simulink model "uas_main_latest"  (R2025a)
settings: Solver=FixedStepAuto  StartTime=0.0  StopTime=Inf  FixedStep=sample_time  RelTol=1e-3
model workspace: external: MAT-File (data not in the file)
values from neighbouring files (symbols this model uses):
  arm_length = 0.17    [test_uas_parameters.m]    (also in uas_parameters.m; uas_parameters_akin.m; uas_parameters_brushless.m = 0.046)
  drag_coefficient = 0.47    [uas_parameters.m]    (also in uas_parameters_akin.m; uas_parameters_brushless.m)
  g = 9.80665    [test_uas_parameters.m]    (also in uas_parameters.m; uas_parameters_akin.m; uas_parameters_brushless.m)
  inertia_xx = 0.007    [test_uas_parameters.m]    (also in uas_parameters.m; uas_parameters_akin.m; uas_parameters_brushless.m = 1.657171e-05)
  inertia_yy = 0.007    [test_uas_parameters.m]    (also in uas_parameters.m; uas_parameters_akin.m; uas_parameters_brushless.m = 1.6655602e-05)
  inertia_zz = 0.012    [test_uas_parameters.m]    (also in uas_parameters.m; uas_parameters_akin.m; uas_parameters_brushless.m = 2.9261652e-05)
  mass_drone = 0.68    [test_uas_parameters.m]    (also in uas_parameters.m; uas_parameters_akin.m; uas_parameters_brushless.m = 0.037)
  mass_total = mass_drone    (= 0.68)    [test_uas_parameters.m]    (also in uas_parameters.m; uas_parameters_akin.m; uas_parameters_brushless.m = 0.037)
  max_rot_velocity = 838    [uas_parameters.m]    (also in uas_parameters_akin.m; uas_parameters_brushless.m)
  mix_matrix = inv(motor_constant * allocation_matrix)    [test_uas_parameters.m]    (also in uas_parameters.m; uas_parameters_akin.m; uas_parameters_brushless.m)
  moment_constant = 0.016    [test_uas_parameters.m]    (also in uas_parameters.m; uas_parameters_akin.m; uas_parameters_brushless.m = 0.006)
  motor_constant = 8.54858e-06    [test_uas_parameters.m]    (also in uas_parameters.m; uas_parameters_akin.m; uas_parameters_brushless.m = 1.45e-08)
  publish_rate = sample_time    (= 0.04)    [test_uas_parameters.m]    (also in uas_parameters.m; uas_parameters_akin.m; uas_parameters_brushless.m)
  reference_area = pi * (75e-3)^2    (= 0.0176714586764)    [uas_parameters.m]    (also in uas_parameters_akin.m; uas_parameters_brushless.m)
  rotor_offset_top = 0.01    [uas_parameters.m]    (also in uas_parameters_akin.m; uas_parameters_brushless.m)
  route = route_scaled    [generate_route_for_simulink.m]    (also in uas_parameters.m = route_smooth; uas_parameters_akin.m = route_dense; uas_parameters_brushless.m = [0 0 1 ; 9 0 1 ; 9 9 1])
  sample_time = 4e-2    (= 0.04)    [test_uas_parameters.m]    (also in uas_parameters.m; uas_parameters_akin.m; uas_parameters_brushless.m)
  x0 = route_world(1,1)    [uas_parameters.m]    (also in uas_parameters_akin.m = route(1,1); uas_parameters_brushless.m = 36)
  y0 = route_world(1,2)    [uas_parameters.m]    (also in uas_parameters_akin.m = route(1,2); uas_parameters_brushless.m = 80)
  z0 = route_world(1,3)    [uas_parameters.m]    (also in uas_parameters_akin.m = route(1,3); uas_parameters_brushless.m = 1)
undefined symbols (not defined in the file or in its folder): Angular, Linear, poly_traj, Position, quat2rotm, X, Y, Z
libraries: nesl_utility x32, sm_lib x25, ros2lib x8, sim3dlib x1, uavsim3dlib x1, simulink x1, vrlib x1, simulink_extras x1
(part 1 of 2)
settings Model: Creator=david  LastModifiedBy=rami
settings SolverCC: AlgebraicLoopSolver=TrustRegion
settings DataIOCC: LimitDataPoints=on  MaxDataPoints=10000
settings OptimizationCC: EnhancedBackFolding=on  PassReuseOutputArgsThreshold=0.0  ZeroExternalMemoryAtStartup=off  ZeroInternalMemoryAtStartup=off  MaxStackSize=64  OptimizeBlockOrder=speed  DifferentSizesBufferReuse=on  OptimizationCustomize=off
settings DebuggingCC: ParameterTunabilityLossMsg=error  UnconnectedInputMsg=warning  UnconnectedOutputMsg=warning  UnconnectedLineMsg=warning  AllowSymbolicDim=off  SFUnexpectedBacktrackingDiag=warning  SFNoUnconditionalDefaultTransitionDiag=warning  SFExecutionAtInitializationDiag=none  UnderSpecifiedDimensionMsg=warning  ArithmeticOperatorsInVariantConditions=warning
settings HardwareCC: ProdBitPerPointer=32.0  ProdBitPerSizeT=32.0  ProdBitPerPtrDiffT=32.0  ProdLargestAtomicFloat=None  ProdIntDivRoundTo=Undefined  ProdEndianess=Unspecified  ProdWordSize=32.0  ProdHWDeviceType=Generic->Unspecified (assume 32-bit Generic)  UseEmbeddedCoderFeatures=off
settings ModelReferenceCC: EnableRefExpFcnMdlSchedulingChecks=on
settings SFSimCC: SimUseLocalCustomCode=off  MATLABDynamicMemAlloc=off  CustomCodeUndefinedFunction=UseInterfaceOnly  SimTargetLang=C++  SimDLTargetLibrary=mkl-dnn
settings RTWCC: SystemTargetFile=ert.tlc  HardwareBoard=Robot Operating System (ROS)  TLCOptions="-aInlineSetEventsForThisBaseRateFcn=TLC_FALSE -aSuppressMultiTaskScheduler=TLC_FALSE  -aRateBasedStepFcn=0"  GenCodeOnly=on  TemplateMakefile=ert_default_tmf  RTWUseLocalCustomCode=off  Toolchain=Catkin  TargetLang=C++  GPUComputeCapability=3.5  DLArmComputeVersion=19.05  Description=Embedded Coder
settings CodeAppCC: ForceParamTrailComments=on  OperatorAnnotations=on
settings ERTTargetCC: ExtModeTransport=0.0  ExtModeStaticAlloc=off  ExtModeMexFile=ext_comm  ExtModeIntrfLevel=Level1  InlinedParameterPlacement=Hierarchical  RootIOFormat=Structure reference  DynamicArrayContainerType=coder::array  ERTCustomFileBanners=off  CodeInterfacePackaging=C++ class  SupportContinuousTime=on  SupportNonInlinedSFcns=on  RemoveResetFunc=off  ModelStepFunctionPrototypeControlCompliant=off
settings ConfigComp: CovMetricSettings=dw  CovSaveCumulativeToWorkspaceVar=on  CovSaveSingleToWorkspaceVar=on  CovExternalEMLEnable=off  CovSFcnEnable=off
settings SimscapeCC: SimscapeLogType=all  SimscapeLogSimulationStatistics=on  SimscapeLogDataHistory=10000.0
settings ExplorerConfigSet: InternalSimMechanicsExplorerSettings="<ExplorerConfiguration><canonicalview>default</canonicalview><AnimationSetting><BasePlaybackSpeed>1.0</BasePlaybackSpeed><PlaybackSpeedFactor>1.0</PlaybackSpeedFactor></AnimationSetting><TilePanel><TileInfo><Tiles Columns=\"1\" Count=\"1\" Rows=\"1\"><Column Weight=\"1\"/><Row Weight=\"1\"/><Tile Height=\"1\" Width=\"1\" X=\"0\" Y=\"0\"/></Tiles></TileInfo><SceneInfo><SceneViewer><BGColor><R>0.400000005960464478</R><G>0.400000005960464478</G><B>0.400000005960464478</B></BGColor><Camera><DoPerspective>off</DoPerspective><Position><X>7.41918867546502359</X><Y>0.562842449888731333</Y><Z>8.36768126399918444</Z></Position><Center><X>4.24878770726833288</X><Y>4.27540210027623324</Y><Z>0.996100590645515815</Z></Center><Up><X>-0.578313069199200891</X><Y>0.601173295476169489</Y><Z>0.551493121262380703</Z></Up><ViewLimDist>1</ViewLimDist><YLim>5.48746925830841104</YLim><XLim>8.41878250057976274</XLim></Camera></SceneViewer></SceneInfo></TilePanel><MechEditorPanel><Cameras/><GfxPanelCameraMap/><VideoCreator><PlaybackSpeedRatio>1.0</PlaybackSpeedRatio><FrameRate>30</FrameRate><VideoFormat>Motion JPEG AVI</VideoFormat><FrameSize>auto</FrameSize></VideoCreator></MechEditorPanel></ExplorerConfiguration>"

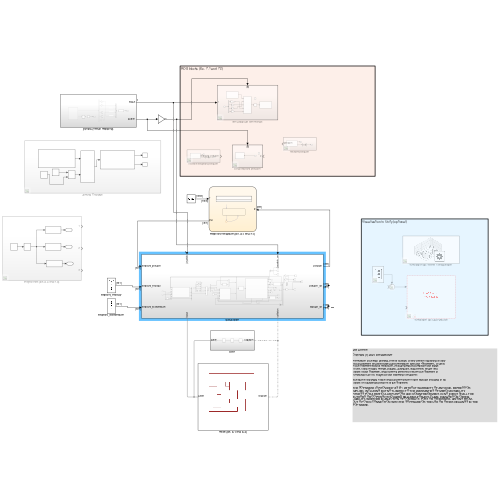
[thumbnail: Simulink's stored preview of the top-level diagram]
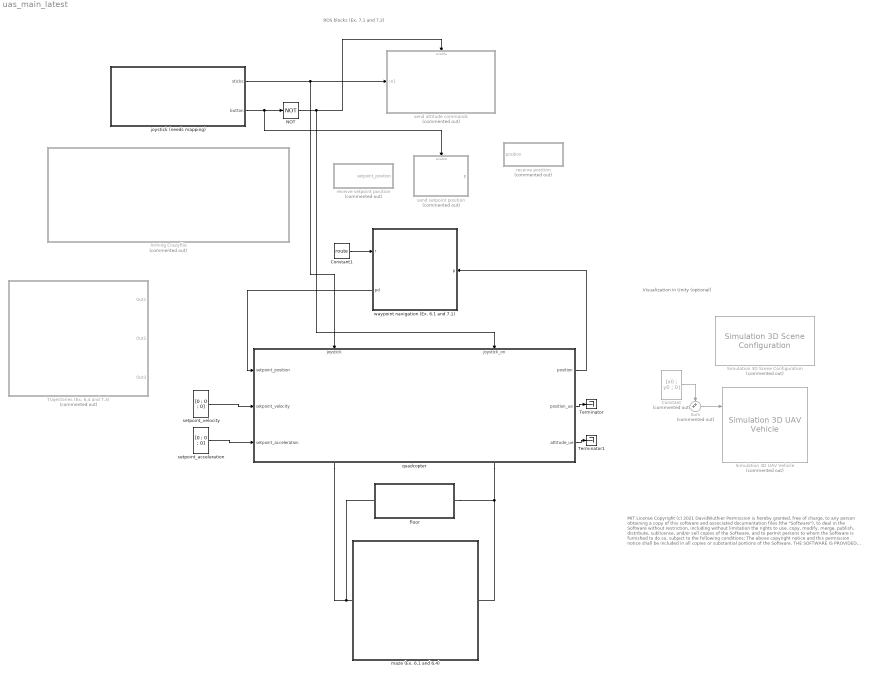
== system uas_main_latest ==
  note: MIT License
      |
      | Copyright (c) 2021 DavidWuthier
      |
      | Permission is hereby granted, free of charge, to any person obtaining a copy
      | of this software and associated documentation files (the "Software"), to deal
      | in the Software without restriction, including without limitation the rights
      | to use, copy, modify, merge, publish, distribute, sublicense, and/or sell
      | copies of the Software, and to permit persons to whom the Software is
      | furnished to do so, subject to the following conditions:
      |
      | The above copyright notice and this permission notice shall be included in all
      | copies or substantial portions of the Software.
      |
      | THE SOFTWARE IS PROVIDED "AS IS", WITHOUT WARRANTY OF ANY KIND, EXPRESS OR
      | IMPLIED, INCLUDING BUT NOT LIMITED TO THE WARRANTIES OF MERCHANTABILITY,
      | FITNESS FOR A PARTICULAR PURPOSE AND NONINFRINGEMENT. IN NO EVENT SHALL THE
      | AUTHORS OR COPYRIGHT HOLDERS BE LIABLE FOR ANY CLAIM, DAMAGES OR OTHER
      | LIABILITY, WHETHER IN AN ACTION OF CONTRACT, TORT OR OTHERWISE, ARISING FROM,
      | OUT OF OR IN CONNECTION WITH THE SOFTWARE OR THE USE OR OTHER DEALINGS IN THE
      | SOFTWARE.
  note: Visualization in Unity (optional)
  note: ROS blocks (Ex. 7.1 and 7.2)
  Arming Crazyflie : Subsystem  Commented=on
  Constant : Constant  Commented=on  Value=[x0 ; y0 ; 0]  VectorParams1D=off
  Constant1 : Constant  Value=route
  NOT : Logic  Operator=NOT  IconShape=distinctive  AllPortsSameDT=off  OutDataTypeStr=boolean
  Simulation 3D Scene Configuration : sim3dlib/Simulation 3D Scene Configuration  Priority=0  Commented=on  ProjectFormat=Default Scenes  SceneDesc=US city block  ProjectName=/usr/local/MATLAB/R2025a/toolbox/shared/sim3d_projects/automotive_project_linux/UE/LinuxNoEditor/VehicleSimulation.sh  ScenePath=/Game/Maps/USCityBlock  EnableOpenDRIVE=off  vehTagList={'Scene Origin';'SimulinkVehicle1'}  vehTag=SimulinkVehicle1  AttachedCameraRelativeTranslation=[0 0 0]  FreeCameraDefaultInitialTranslation=[-6, 0, 2]  AttachedCameraRelativeRotation=[0 0 0]  FreeCameraDefaultInitialRotation=[0, -15, 0]  ViewpointName=Custom  FreeCameraInitialTranslation=[0, 0, 0]  ViewpointTranslation=[0 0 0]  FreeCameraInitialRotation=[0, 0, 0]  ViewpointRotation=[0 0 0]  OpVisEn=off  Ts=sample_time  EnableWindow=on  EnableRemoteAccess=off  EnableWeather=off  SunAzimuth=90  SunAltitude=40.0  EnableGeospatialSun=off  Latitude=0  Longitude=0  Date=2023-01-01  Time=10:30:00  GeoTimeZone=-5.0  SunDaylightSaving=off  wind=1  clouds=10  EnableVolumetricClouds=off  CloudCoverage=0  CloudAltitude=6  fog=0  rain=0  RaindropsEffect=off  SnowDensity=0  EnableGeospatial=off  TilesetSource=Earth terrain  UseTrueOrigin=off  OriginHeight=200  OriginLatitude=40.744652  OriginLongitude=-73.988864  MapStyle=Aerial  AdditionalAssetIDs=[]  UseAdvancedSunSky=off  SolarTime=11  TimeZone=-5  Day=21  Month=9  Year=2022  UseDaylightSavingTime=on  DSTStartDay=10  DSTStartMonth=3  DSTEndDay=3  DSTEndMonth=11  DSTSwitchHour=2  sensorTag=MainCamera1  sensorId=1  sensorName=MainCamera1  mountLoc=Origin  offsetFlag=off  tmountOffset=[0, 0, 0]  rmountOffset=[0, 0, 0]  HorizontalResolution=1280  VerticalResolution=720  HorizontalFOV=60  mountPoint=[0 0 0]  mountOrientation=[0 0 0]  aMode=4  ID=1  GeoTrigger=Inactive  ViewNameList={'Custom'}  ViewTranslationList={'[0 0 0]'}  ViewRotationList={'[0 0 0]'}
      settings: LibrarySourceBlock=uavsim3dlib/Simulation 3D Scene Configuration
  Simulation 3D UAV Vehicle : uavsim3dlib/Simulation 3D UAV Vehicle  Commented=on  Mesh=Quadrotor  MeshPath=/MathWorksUAVContent/UAVs/HexaRotorUAV/HexaRotor.HexaRotor  Color=Black  ActorName=SimulinkVehicle1  UseGlobalFrame=off  InitialTranslation=[x0 y0 z0]  InitialRotation=[0 0 0]  InitialTranslationGlobal=[0 0 0]  InitialGeoOrigin=[0 0 0]  InitialRotationGlobal=[0 0 0]  SampleTime=-1  ActorType=SimulinkVehicle  ID=1  aMode=4  ActorTag=SimulinkVehicle1
  Sum : Sum  Commented=on  Inputs=++|
  Terminator : Terminator
  Terminator1 : Terminator
  Trajectories (Ex. 6.4 and 7.3) : Subsystem  Commented=on
  floor : Subsystem
  joystick (needs mapping) : Subsystem
  maze (Ex. 6.1 and 6.4) : Subsystem
      mask Display: image('$imagefile'); % Use "Edit Image" on toolstrip to change.
  quadcopter : Subsystem
      settings: PortSchema="{\"entries\":[{\"content\":{\"sides\":[{\"content\":{\"connectorIds\":[\"In1\",\"In2\",\"In3\"]},\"type\":\"ConnectorPlacement.EquallySpacedRectSide\",\"uuid\":\"ed16c4a7-5f5f-48d5-8471-b227eef37b0b\"},{\"content\":{\"connectorIds\":[\"Out1\",\"Out2\",\"Out3\"],\"side\":\"RIGHT\"},\"type\":\"ConnectorPlacement.EquallySpacedRectSide\",\"uuid\":\"303ea24f-0a15-469a-b5d8-cc8b33d29b5f\"},{\"content\":{\"connectorIds\":[\"In4\",\"In5\"],\"side\":\"TOP\"},\"type\":\"ConnectorPlacement.EquallySpacedRectSide\",\"uuid\":\"d3970502-0872-434b-b7c5-387e72ad4178\"},{\"content\":{\"connectorIds\":[\"RConn1\",\"RConn2\"],\"side\":\"BOTTOM\"},\"type\":\"ConnectorPlacement.EquallySpacedRectSide\",\"uuid\":\"dd808c8e-2f91-44fb-8d51-5dec3bd81dd9\"}]},\"type\":\"ConnectorPlacement.EquallySpacedConnector\",\"uuid\":\"aacf4a84-08b7-4fd3-a02a-51c4e2a4df71\"}],\"packageUris\":[\"http://schema.mathworks.com/mf0/Connector/R2020b\"],\"version\":\"1.0\"}"
  receive position : Subsystem  Commented=on
  receive setpoint position : Subsystem  Commented=on
  send attitude commands : Subsystem  Commented=on
  send setpoint position : Subsystem  Commented=on
  setpoint_acceleration : Constant  Value=[0 ; 0 ; 0]  VectorParams1D=off
  setpoint_velocity : Constant  Value=[0 ; 0 ; 0]  VectorParams1D=off
  waypoint navigation (Ex. 6.1 and 7.1) : Stateflow chart  TreatAsAtomicUnit=on
      settings: PortSchema="{\"entries\":[{\"content\":{\"sides\":[{\"content\":{\"connectorIds\":[\"In1\",\"Out1\"]},\"type\":\"ConnectorPlacement.EquallySpacedRectSide\",\"uuid\":\"7c2fff0d-1179-4786-9432-1971d7acd904\"},{\"content\":{\"connectorIds\":[\"In2\"],\"side\":\"RIGHT\"},\"type\":\"ConnectorPlacement.EquallySpacedRectSide\",\"uuid\":\"377a8206-b310-41c0-9a17-faf5318c89cb\"},{\"content\":{\"side\":\"TOP\"},\"type\":\"ConnectorPlacement.EquallySpacedRectSide\",\"uuid\":\"b953090a-ffdb-4e30-a5fe-7bef9655f1cf\"},{\"content\":{\"side\":\"BOTTOM\"},\"type\":\"ConnectorPlacement.EquallySpacedRectSide\",\"uuid\":\"03dc7a24-529e-4020-b953-d1c4751c5c80\"}]},\"type\":\"ConnectorPlacement.EquallySpacedConnector\",\"uuid\":\"03bac9f4-6480-492d-9af3-57aec4db8fd8\"}],\"packageUris\":[\"http://schema.mathworks.com/mf0/Connector/R2020b\"],\"version\":\"1.0\"}"
  wires:
  Sum/1 -> Simulation 3D UAV Vehicle/1
  Constant/1 -> Sum/1
  Constant1/1 -> waypoint navigation (Ex. 6.1 and 7.1)/1(r)
  setpoint_velocity/1 -> quadcopter/2(setpoint_velocity)
  setpoint_acceleration/1 -> quadcopter/3(setpoint_acceleration)
  NOT/1 -> quadcopter/5(joystick_on), send attitude commands/Enable
  joystick (needs mapping)/1(sticks) -> send attitude commands/1(In1), quadcopter/4(joystick)
  joystick (needs mapping)/2(button) -> NOT/1, send setpoint position/Enable
  quadcopter/1(position) -> waypoint navigation (Ex. 6.1 and 7.1)/2(p)
  waypoint navigation (Ex. 6.1 and 7.1)/1(pd) -> quadcopter/1(setpoint_position)
  quadcopter/2(position_ue) -> Terminator/1
  quadcopter/3(attitude_ue) -> Terminator1/1
  connections:
  floor/LConn1 -- quadcopter/RConn1 -- maze (Ex. 6.1 and 6.4)/LConn1
  floor/RConn1 -- quadcopter/RConn2 -- maze (Ex. 6.1 and 6.4)/RConn1

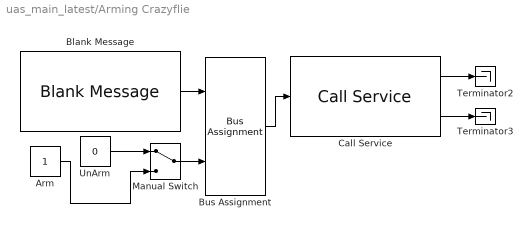
== system uas_main_latest/Arming Crazyflie ==
  Arm : Constant  OutDataTypeStr=boolean
  Blank Message : ros2lib/Blank Message  messageClass=Service Request  entityType=crazyflie_interfaces/Arm  messageType=crazyflie_interfaces/ArmRequest  SampleTime=inf
  Bus Assignment : BusAssignment  AssignedSignals=arm
  Call Service : ros2lib/Call Service  topicSource=Specify your own  service=/cf231/arm  serviceType=crazyflie_interfaces/Arm  connectionTimeout=5  ShowErrorCodeOutput=on  legacyBusStruct=off  QOSHistory=Keep last  QOSDepth=1  QOSReliability=Reliable  QOSDurability=Volatile  QOSDeadline=Inf  QOSLifespan=Inf  QOSLiveliness=Automatic  QOSLeaseDuration=Inf  QOSAvoidROSNamespaceConventions=off
  Manual Switch : ManualSwitch
  Terminator2 : Terminator
  Terminator3 : Terminator
  UnArm : Constant  Value=0  OutDataTypeStr=boolean
  wires:
  Blank Message/1 -> Bus Assignment/1
  UnArm/1 -> Manual Switch/1
  Arm/1 -> Manual Switch/2
  Call Service/1 -> Terminator2/1
  Bus Assignment/1 -> Call Service/1
  Manual Switch/1 -> Bus Assignment/2
  Call Service/2 -> Terminator3/1

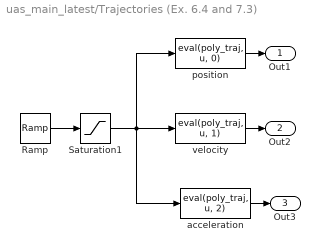
== system uas_main_latest/Trajectories (Ex. 6.4 and 7.3) ==
  Ramp : simulink/Sources/Ramp  slope=1  start=0  InitialOutput=0
  Saturation1 : Saturate  UpperLimit=knots(end)  LowerLimit=0
  acceleration : MATLABFcn  MATLABFcn=eval(poly_traj, u, 2)  OutputDimensions=[3 1]  Output1D=off
  position : MATLABFcn  MATLABFcn=eval(poly_traj, u, 0)  OutputDimensions=[3 1]  Output1D=off
  velocity : MATLABFcn  MATLABFcn=eval(poly_traj, u, 1)  OutputDimensions=[3 1]  Output1D=off
  Out1 : Outport
  Out2 : Outport  Port=2
  Out3 : Outport  Port=3
  wires:
  Saturation1/1 -> acceleration/1, position/1, velocity/1
  Ramp/1 -> Saturation1/1
  velocity/1 -> Out2/1
  position/1 -> Out1/1
  acceleration/1 -> Out3/1

== system uas_main_latest/floor ==
  Brick Solid1 : sm_lib/Body Elements/Brick Solid  BrickDimensions=[3 3 0.1]  BrickDimensionsUnits=m  ExportEntireGeometry=on  InertiaType=CalculateFromGeometry  BasedOnType=Density  Density=0  DensityUnits=kg/m^3  Mass=1  MassUnits=kg  CenterOfMass=[0 0 0]  CenterOfMassUnits=m  MomentsOfInertia=[1 1 1]  MomentsOfInertiaUnits=kg*m^2  ProductsOfInertia=[0 0 0]  ProductsOfInertiaUnits=kg*m^2  GraphicType=FromGeometry  MarkerShape=Sphere  MarkerSize=10  GraphicVisPropType=SimpleVisualProperties  GraphicDiffuseColor=[0.4 0.4 0.4]  GraphicOpacity=1  GraphicSpecularColor=[0.5 0.5 0.5 1.0]  GraphicAmbientColor=[0.15 0.15 0.15 1.0]  GraphicEmissiveColor=[0.0 0.0 0.0 1.0]  GraphicShininess=75  DoExposeReferenceFrame=on  SerializedFrames=<Frames/>
  Rigid Transform5 : sm_lib/Frames and Transforms/Rigid Transform  RotationMethod=None  FollAlignAxisA=+X  BaseAlignAxisA=+Y  FollAlignAxisB=+Y  BaseAlignAxisB=+Z  RotationStandardAxis=+Z  RotationAngle=0.0  RotationAngleUnits=deg  RotationArbitraryAxis=[0 0 1]  RotationSequenceAxes=FollowerAxes  RotationSequence=XYX  RotationSequenceAngles=[0 0 0]  RotationSequenceAnglesUnits=deg  RotationMatrix=[1 0 0; 0 1 0; 0 0 1]  Quaternion=[1 0 0 0]  TranslationMethod=StandardAxis  TranslationCartesianOffset=[0 0 0]  TranslationCartesianOffsetUnits=m  TranslationStandardAxis=-Z  TranslationStandardOffset=0.05  TranslationStandardOffsetUnits=m  TranslationROffset=0  TranslationROffsetUnits=m  TranslationThetaOffset=0  TranslationThetaOffsetUnits=deg  TranslationZOffset=0  TranslationZOffsetUnits=m
  Spatial Contact Force : sm_lib/Forces and Torques/Spatial Contact Force  SenseSeparationDistance=off  NormalForceType=SmoothSpringDamper  NormalStiffness=stiffness_wall  NormalStiffnessUnits=N/m  NormalDamping=critical_damping_wall  NormalDampingUnits=N/(m/s)  NormalTransitionRegionWidth=1e-4  NormalTransitionRegionWidthUnits=m  FrictionType=SmoothStickSlip  CoefficientOfStaticFriction=0.5  CoefficientOfDynamicFriction=0.3  FrictionalCriticalVelocity=1e-3  FrictionalCriticalVelocityUnits=m/s  SenseContactSignal=off  SensePenetrationDepth=off  SenseNormalVelocity=off  SenseTangentialVelocity=off  SensingForceTorqueDirection=BaseOnFollower  SensingForceTorqueResolutionFrame=ContactFrame  SenseNormalForce=off  SenseNormalForceMagnitude=off  SenseNormalTorque=off  SenseFrictionalForce=off  SenseFrictionalForceMagnitude=off  SenseFrictionalTorque=off  SenseTotalForce=off  SenseTotalTorque=off  SenseContactBaseRotation=off  SenseContactBaseTranslation=off  SenseContactFollowerRotation=off  SenseContactFollowerTranslation=off  ZeroCrossDetectContactStartAndEnd=off
  base : PMIOPort  Side=Left
  collision : PMIOPort  Port=2  Side=Right
  connections:
  Rigid Transform5/RConn1 -- Brick Solid1/RConn1
  Rigid Transform5/LConn1 -- base/RConn1
  Spatial Contact Force/RConn1 -- Brick Solid1/LConn1
  Spatial Contact Force/LConn1 -- collision/RConn1

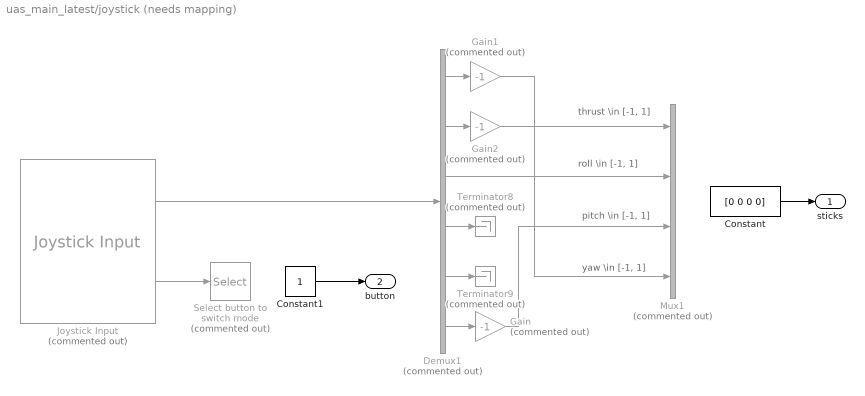
== system uas_main_latest/joystick (needs mapping) ==
  note: thrust \in [-1, 1]
  note: roll \in [-1, 1]
  note: pitch \in [-1, 1]
  note: yaw \in [-1, 1]
  Constant : Constant  Value=[0 0 0 0]
  Constant1 : Constant
  Demux1 : Demux  Commented=on  Outputs=6
  Gain : Gain  Commented=on  Gain=-1
  Gain1 : Gain  Commented=on  Gain=-1
  Gain2 : Gain  Commented=on  Gain=-1
  Joystick Input : vrlib/Joystick Input  Commented=on  joyid=1  adjustports=on  forcefeed=off
  Mux1 : Mux  Commented=on
  Select button to switch mode : Selector  Commented=on  InputPortWidth=15  IndexOptions=Index vector (dialog)  Indices=8  OutputSizes=1
  Terminator8 : Terminator  Commented=on
  Terminator9 : Terminator  Commented=on
  sticks : Outport
  button : Outport  Port=2
  wires:
  Gain1/1 -> Mux1/4
  Joystick Input/1 -> Demux1/1
  Gain2/1 -> Mux1/1
  Demux1/1 -> Gain1/1
  Joystick Input/2 -> Select button to switch mode/1
  Demux1/6 -> Gain/1
  Demux1/5 -> Terminator9/1
  Demux1/3 -> Mux1/2
  Demux1/2 -> Gain2/1
  Demux1/4 -> Terminator8/1
  Gain/1 -> Mux1/3
  Constant/1 -> sticks/1
  Constant1/1 -> button/1

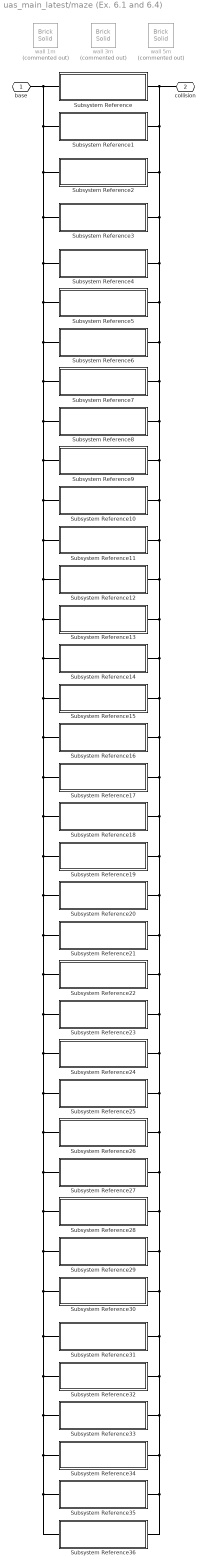
== system uas_main_latest/maze (Ex. 6.1 and 6.4) ==
  Subsystem Reference : Subsystem  ReferencedSubsystem=uas_wall  l=5  x=-1  y=1.5  yaw=0
  Subsystem Reference1 : Subsystem  ReferencedSubsystem=uas_wall  l=5  x=-1  y=7.5  yaw=0
  Subsystem Reference10 : Subsystem  ReferencedSubsystem=uas_wall  l=5  x=7.5  y=10  yaw=pi/2
  Subsystem Reference11 : Subsystem  ReferencedSubsystem=uas_wall  l=5  x=5  y=10  yaw=pi/2
  Subsystem Reference12 : Subsystem  ReferencedSubsystem=uas_wall  l=5  x=1.5  y=1  yaw=pi/2
  Subsystem Reference13 : Subsystem  ReferencedSubsystem=uas_wall  l=3  x=4.5  y=1  yaw=pi/2
  Subsystem Reference14 : Subsystem  ReferencedSubsystem=uas_wall  l=3  x=8  y=2.5  yaw=0
  Subsystem Reference15 : Subsystem  ReferencedSubsystem=uas_wall  l=1  x=6  y=4.5  yaw=0
  Subsystem Reference16 : Subsystem  ReferencedSubsystem=uas_wall  l=1  x=6  y=1.5  yaw=0
  Subsystem Reference17 : Subsystem  ReferencedSubsystem=uas_wall  l=1  x=2  y=1.5  yaw=0
  Subsystem Reference18 : Subsystem  ReferencedSubsystem=uas_wall  l=1  x=0  y=2.5  yaw=0
  Subsystem Reference19 : Subsystem  ReferencedSubsystem=uas_wall  l=5  x=5.5  y=4  yaw=pi/2
  Subsystem Reference2 : Subsystem  ReferencedSubsystem=uas_wall  l=5  x=-1  y=5  yaw=0
  Subsystem Reference20 : Subsystem  ReferencedSubsystem=uas_wall  l=1  x=4  y=3.5  yaw=0
  Subsystem Reference21 : Subsystem  ReferencedSubsystem=uas_wall  l=1  x=2.5  y=4  yaw=pi/2
  Subsystem Reference22 : Subsystem  ReferencedSubsystem=uas_wall  l=1  x=0.5  y=2  yaw=pi/2
  Subsystem Reference23 : Subsystem  ReferencedSubsystem=uas_wall  l=1  x=1.5  y=2  yaw=pi/2
  Subsystem Reference24 : Subsystem  ReferencedSubsystem=uas_wall  l=1  x=-0.5  y=3  yaw=pi/2
  Subsystem Reference25 : Subsystem  ReferencedSubsystem=uas_wall  l=1  x=2  y=4.5  yaw=0
  Subsystem Reference26 : Subsystem  ReferencedSubsystem=uas_wall  l=1  x=1.5  y=5  yaw=pi/2
  Subsystem Reference27 : Subsystem  ReferencedSubsystem=uas_wall  l=1  x=0.5  y=7  yaw=pi/2
  Subsystem Reference28 : Subsystem  ReferencedSubsystem=uas_wall  l=1  x=1  y=7.5  yaw=0
  Subsystem Reference29 : Subsystem  ReferencedSubsystem=uas_wall  l=2  x=8  y=7  yaw=0
  Subsystem Reference3 : Subsystem  ReferencedSubsystem=uas_wall  l=5  x=10  y=1.5  yaw=0
  Subsystem Reference30 : Subsystem  ReferencedSubsystem=uas_wall  l=1  x=-0.5  y=7  yaw=pi/2
  Subsystem Reference31 : Subsystem  ReferencedSubsystem=uas_wall  l=1  x=6  y=5.5  yaw=0
  Subsystem Reference32 : Subsystem  ReferencedSubsystem=uas_wall  l=5  x=5.5  y=8  yaw=pi/2
  Subsystem Reference33 : Subsystem  ReferencedSubsystem=uas_wall  l=1  x=3.5  y=7  yaw=pi/2
  Subsystem Reference34 : Subsystem  ReferencedSubsystem=uas_wall  l=1  x=3  y=7.5  yaw=0
  Subsystem Reference35 : Subsystem  ReferencedSubsystem=uas_wall  l=1  x=4  y=6.5  yaw=0
  Subsystem Reference36 : Subsystem  ReferencedSubsystem=uas_wall  l=1  x=4  y=7.5  yaw=0
  Subsystem Reference4 : Subsystem  ReferencedSubsystem=uas_wall  l=5  x=10  y=7.5  yaw=0
  Subsystem Reference5 : Subsystem  ReferencedSubsystem=uas_wall  l=5  x=10  y=5  yaw=0
  Subsystem Reference6 : Subsystem  ReferencedSubsystem=uas_wall  l=5  x=1.5  y=-1  yaw=pi/2
  Subsystem Reference7 : Subsystem  ReferencedSubsystem=uas_wall  l=5  x=7.5  y=-1  yaw=pi/2
  Subsystem Reference8 : Subsystem  ReferencedSubsystem=uas_wall  l=5  x=5  y=-1  yaw=pi/2
  Subsystem Reference9 : Subsystem  ReferencedSubsystem=uas_wall  l=5  x=1.5  y=10  yaw=pi/2
  wall 1m : sm_lib/Body Elements/Brick Solid  Commented=on  BrickDimensions=[0.1 1 2]  BrickDimensionsUnits=m  ExportEntireGeometry=on  InertiaType=CalculateFromGeometry  BasedOnType=Density  Density=1000  DensityUnits=kg/m^3  Mass=1  MassUnits=kg  CenterOfMass=[0 0 0]  CenterOfMassUnits=m  MomentsOfInertia=[1 1 1]  MomentsOfInertiaUnits=kg*m^2  ProductsOfInertia=[0 0 0]  ProductsOfInertiaUnits=kg*m^2  GraphicType=FromGeometry  MarkerShape=Sphere  MarkerSize=10  GraphicVisPropType=SimpleVisualProperties  GraphicDiffuseColor=wall_color  GraphicOpacity=1.0  GraphicSpecularColor=[0.5 0.5 0.5 1.0]  GraphicAmbientColor=[0.15 0.15 0.15 1.0]  GraphicEmissiveColor=[0.0 0.0 0.0 1.0]  GraphicShininess=75  DoExposeReferenceFrame=on  SerializedFrames=<Frames/>
  wall 3m : sm_lib/Body Elements/Brick Solid  Commented=on  BrickDimensions=[0.1 3 2]  BrickDimensionsUnits=m  ExportEntireGeometry=on  InertiaType=CalculateFromGeometry  BasedOnType=Density  Density=1000  DensityUnits=kg/m^3  Mass=1  MassUnits=kg  CenterOfMass=[0 0 0]  CenterOfMassUnits=m  MomentsOfInertia=[1 1 1]  MomentsOfInertiaUnits=kg*m^2  ProductsOfInertia=[0 0 0]  ProductsOfInertiaUnits=kg*m^2  GraphicType=FromGeometry  MarkerShape=Sphere  MarkerSize=10  GraphicVisPropType=SimpleVisualProperties  GraphicDiffuseColor=wall_color  GraphicOpacity=1.0  GraphicSpecularColor=[0.5 0.5 0.5 1.0]  GraphicAmbientColor=[0.15 0.15 0.15 1.0]  GraphicEmissiveColor=[0.0 0.0 0.0 1.0]  GraphicShininess=75  DoExposeReferenceFrame=on  SerializedFrames=<Frames/>
  wall 5m : sm_lib/Body Elements/Brick Solid  Commented=on  BrickDimensions=[0.1 5 2]  BrickDimensionsUnits=m  ExportEntireGeometry=on  InertiaType=CalculateFromGeometry  BasedOnType=Density  Density=1000  DensityUnits=kg/m^3  Mass=1  MassUnits=kg  CenterOfMass=[0 0 0]  CenterOfMassUnits=m  MomentsOfInertia=[1 1 1]  MomentsOfInertiaUnits=kg*m^2  ProductsOfInertia=[0 0 0]  ProductsOfInertiaUnits=kg*m^2  GraphicType=FromGeometry  MarkerShape=Sphere  MarkerSize=10  GraphicVisPropType=SimpleVisualProperties  GraphicDiffuseColor=wall_color  GraphicOpacity=1.0  GraphicSpecularColor=[0.5 0.5 0.5 1.0]  GraphicAmbientColor=[0.15 0.15 0.15 1.0]  GraphicEmissiveColor=[0.0 0.0 0.0 1.0]  GraphicShininess=75  DoExposeReferenceFrame=on  SerializedFrames=<Frames/>
  base : PMIOPort  Side=Left
  collision : PMIOPort  Port=2  Side=Right
  connections:
  Subsystem Reference35/LConn1 -- Subsystem Reference36/LConn1 -- base/RConn1 -- Subsystem Reference/LConn1 -- Subsystem Reference1/LConn1 -- Subsystem Reference2/LConn1 -- Subsystem Reference3/LConn1 -- Subsystem Reference4/LConn1 -- Subsystem Reference5/LConn1 -- Subsystem Reference6/LConn1 -- Subsystem Reference7/LConn1 -- Subsystem Reference8/LConn1 -- Subsystem Reference9/LConn1 -- Subsystem Reference10/LConn1 -- Subsystem Reference11/LConn1 -- Subsystem Reference12/LConn1 -- Subsystem Reference13/LConn1 -- Subsystem Reference14/LConn1 -- Subsystem Reference15/LConn1 -- Subsystem Reference16/LConn1 -- Subsystem Reference17/LConn1 -- Subsystem Reference18/LConn1 -- Subsystem Reference19/LConn1 -- Subsystem Reference20/LConn1 -- Subsystem Reference21/LConn1 -- Subsystem Reference22/LConn1 -- Subsystem Reference23/LConn1 -- Subsystem Reference24/LConn1 -- Subsystem Reference25/LConn1 -- Subsystem Reference26/LConn1 -- Subsystem Reference27/LConn1 -- Subsystem Reference28/LConn1 -- Subsystem Reference29/LConn1 -- Subsystem Reference30/LConn1 -- Subsystem Reference31/LConn1 -- Subsystem Reference32/LConn1 -- Subsystem Reference33/LConn1 -- Subsystem Reference34/LConn1
  Subsystem Reference32/RConn1 -- Subsystem Reference36/RConn1 -- Subsystem Reference35/RConn1 -- Subsystem Reference34/RConn1 -- Subsystem Reference33/RConn1 -- collision/RConn1 -- Subsystem Reference/RConn1 -- Subsystem Reference1/RConn1 -- Subsystem Reference2/RConn1 -- Subsystem Reference3/RConn1 -- Subsystem Reference4/RConn1 -- Subsystem Reference5/RConn1 -- Subsystem Reference6/RConn1 -- Subsystem Reference7/RConn1 -- Subsystem Reference8/RConn1 -- Subsystem Reference9/RConn1 -- Subsystem Reference10/RConn1 -- Subsystem Reference11/RConn1 -- Subsystem Reference12/RConn1 -- Subsystem Reference13/RConn1 -- Subsystem Reference14/RConn1 -- Subsystem Reference15/RConn1 -- Subsystem Reference16/RConn1 -- Subsystem Reference17/RConn1 -- Subsystem Reference18/RConn1 -- Subsystem Reference19/RConn1 -- Subsystem Reference20/RConn1 -- Subsystem Reference21/RConn1 -- Subsystem Reference22/RConn1 -- Subsystem Reference23/RConn1 -- Subsystem Reference24/RConn1 -- Subsystem Reference25/RConn1 -- Subsystem Reference26/RConn1 -- Subsystem Reference27/RConn1 -- Subsystem Reference28/RConn1 -- Subsystem Reference29/RConn1 -- Subsystem Reference30/RConn1 -- Subsystem Reference31/RConn1

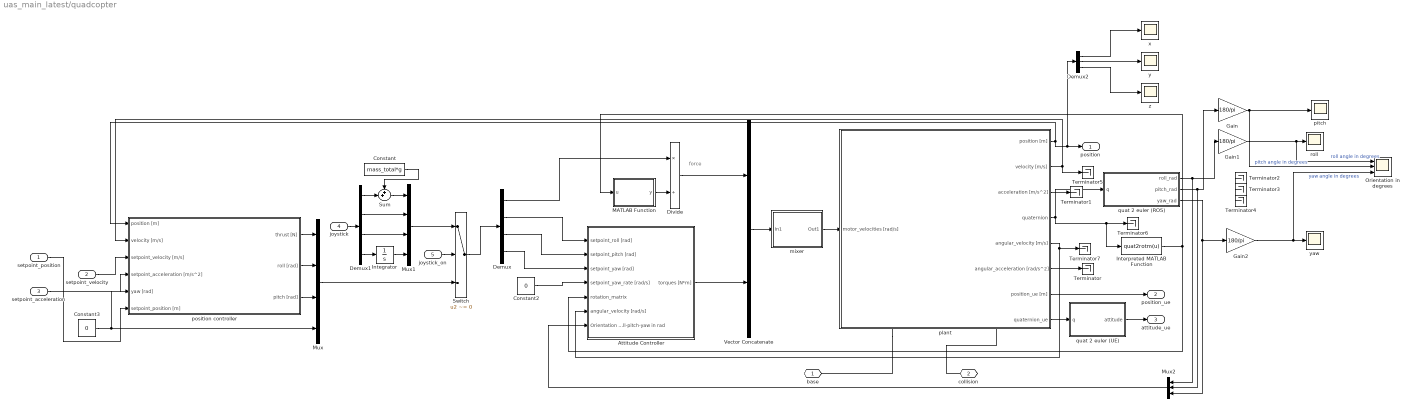
== system uas_main_latest/quadcopter ==
  note: force
  setpoint_position : Inport
  setpoint_velocity : Inport  Port=2
  setpoint_acceleration : Inport  Port=3
  joystick : Inport  Port=4
  joystick_on : Inport  Port=5
  Attitude Controller : Subsystem
      mask Display: image('$imagefile'); % Use "Edit Image" on toolstrip to change.
  Constant : Constant  Value=mass_total*g
  Constant2 : Constant  Value=0
  Constant3 : Constant  Value=0
  Demux : Demux
  Demux1 : Demux
  Demux2 : Demux  Outputs=3
  Divide : Product  Inputs=*/
  Gain : Gain  Gain=180/pi
  Gain1 : Gain  Gain=180/pi
  Gain2 : Gain  Gain=180/pi
  Integrator : Integrator  WrapState=on
  Interpreted MATLAB Function : MATLABFcn  MATLABFcn=quat2rotm(u)  Output1D=off
  MATLAB Function : MATLAB Function  TreatAsAtomicUnit=on
  Mux : Mux
  Mux1 : Mux
  Mux2 : Mux  Inputs=3
  Orientation in degrees : Scope  NumInputPorts=3
      settings: ActiveDisplayYMinimum=-9.05685520240841  ActiveDisplayYMaximum=17.967895493361834  DataLoggingVariableName=ScopeData6
  Sum : Sum  Inputs=++|
  Switch : Switch  Criteria=u2 ~= 0  SaturateOnIntegerOverflow=off  InputSameDT=off
  Terminator{,1..7} (8 alike) : Terminator
  Vector Concatenate : Concatenate
  mixer : Subsystem
  pitch : Scope
      settings: ActiveDisplayYMinimum=-10.74410147910992  ActiveDisplayYMaximum=6.7822864098927491  DataLoggingVariableName=ScopeData9
  plant : Subsystem
      settings: PortSchema="{\"entries\":[{\"content\":{\"sides\":[{\"content\":{\"connectorIds\":[\"In1\"]},\"type\":\"ConnectorPlacement.EquallySpacedRectSide\",\"uuid\":\"6e9c785b-7a58-4a83-84e6-bbea81e0823c\"},{\"content\":{\"connectorIds\":[\"Out1\",\"Out2\",\"Out3\",\"Out4\",\"Out5\",\"Out6\",\"Out7\",\"Out8\"],\"side\":\"RIGHT\"},\"type\":\"ConnectorPlacement.EquallySpacedRectSide\",\"uuid\":\"b008e1e2-aa95-4897-b360-2fe655e93601\"},{\"content\":{\"connectorIds\":[],\"side\":\"TOP\"},\"type\":\"ConnectorPlacement.EquallySpacedRectSide\",\"uuid\":\"363cdb01-a5e5-4a3c-bce9-213e2ffac7b5\"},{\"content\":{\"connectorIds\":[\"RConn1\",\"RConn2\"],\"side\":\"BOTTOM\"},\"type\":\"ConnectorPlacement.EquallySpacedRectSide\",\"uuid\":\"8e0d8754-e9ec-4386-98a0-719833eb7e87\"}]},\"type\":\"ConnectorPlacement.EquallySpacedConnector\",\"uuid\":\"eb300e37-0abf-4331-8664-ac63688da223\"}],\"packageUris\":[\"http://schema.mathworks.com/mf0/Connector/R2020b\"],\"version\":\"1.0\"}"
      mask Display: image('$imagefile'); % Use "Edit Image" on toolstrip to change.
  position controller : Subsystem
      mask Display: image('$imagefile'); % Use "Edit Image" on toolstrip to change.
  quat 2 euler (ROS) : MATLAB Function  TreatAsAtomicUnit=on
  quat 2 euler (UE) : MATLAB Function  TreatAsAtomicUnit=on
  roll : Scope
      settings: ActiveDisplayYMinimum=-0.27365980851842531  ActiveDisplayYMaximum=0.45088677709957792  DataLoggingVariableName=ScopeData3
  x : Scope
      settings: ActiveDisplayYMinimum=-12.039482255836642  ActiveDisplayYMaximum=108.35534030252981
  y : Scope
      settings: ActiveDisplayYMinimum=-0.38012386750282184  ActiveDisplayYMaximum=3.4178941958545219
  yaw : Scope
      settings: ActiveDisplayYMinimum=-0.38484230944438741  ActiveDisplayYMaximum=0.38295623451629723  DataLoggingVariableName=ScopeData4
  z : Scope
      settings: ActiveDisplayYMinimum=-1  ActiveDisplayYMaximum=1  DataLoggingVariableName=ScopeData2
  base : PMIOPort  Side=Right
  collision : PMIOPort  Port=2  Side=Right
  position : Outport
  position_ue : Outport  Port=2
  attitude_ue : Outport  Port=3
  wires:
  plant/4(quaternion) -> Terminator6/1, Interpreted MATLAB Function/1, quat 2 euler (ROS)/1(q)
  plant/6(angular_acceleration [rad/s^2]) -> Terminator/1
  plant/3(acceleration [m/s^2]) -> Terminator1/1
  quat 2 euler (UE)/1(attitude) -> attitude_ue/1
  plant/8(quaternion_ue) -> quat 2 euler (UE)/1(q)
  plant/7(position_ue [m]) -> position_ue/1
  plant/2(velocity [m/s]) -> Terminator5/1, position controller/2(velocity [m/s])
  plant/1(position [m]) -> Demux2/1, position/1, position controller/1(position [m])
  setpoint_acceleration/1 -> position controller/4(setpoint_acceleration [m/s^2])
  setpoint_velocity/1 -> position controller/3(setpoint_velocity [m/s])
  setpoint_position/1 -> position controller/6(setpoint_position [m])
  Constant3/1 -> Mux/4, position controller/5(yaw [rad])
  quat 2 euler (ROS)/1(roll_rad) -> Mux2/1, Gain1/1
  quat 2 euler (ROS)/2(pitch_rad) -> Gain/1, Mux2/2
  position controller/1(thrust [N]) -> Mux/1
  position controller/2(roll [rad]) -> Mux/2
  position controller/3(pitch [rad]) -> Mux/3
  Switch/1 -> Demux/1
  Mux/1 -> Switch/3
  joystick_on/1 -> Switch/2
  joystick/1 -> Demux1/1
  Demux1/2 -> Mux1/2
  Demux1/3 -> Mux1/3
  Mux1/1 -> Switch/1
  Demux1/4 -> Integrator/1
  Integrator/1 -> Mux1/4
  Sum/1 -> Mux1/1
  Constant/1 -> Sum/1
  Demux1/1 -> Sum/2
  Vector Concatenate/1 -> mixer/1(In1)
  mixer/1(Out1) -> plant/1(motor_velocities [rad/s])
  Divide/1 -> Vector Concatenate/1
  Attitude Controller/1(torques [N*m]) -> Vector Concatenate/2
  Interpreted MATLAB Function/1 -> MATLAB Function/1(u), Attitude Controller/5(rotation_matrix)
  Constant2/1 -> Attitude Controller/4(setpoint_yaw_rate [rad/s])
  Demux/4 -> Attitude Controller/3(setpoint_yaw [rad])
  Demux/1 -> Divide/1
  MATLAB Function/1(y) -> Divide/2
  Demux/2 -> Attitude Controller/1(setpoint_roll [rad])
  plant/5(angular_velocity [m/s]) -> Attitude Controller/6(angular_velocity [rad/s]), Terminator7/1
  Demux/3 -> Attitude Controller/2(setpoint_pitch [rad])
  Demux2/2 -> y/1
  Demux2/1 -> x/1
  Demux2/3 -> z/1
  Gain/1 -> Orientation in degrees/2, pitch/1  "pitch angle in degrees"
  Gain1/1 -> Orientation in degrees/1, roll/1  "roll angle in degrees"
  Gain2/1 -> Orientation in degrees/3, yaw/1  "yaw angle in degrees"
  quat 2 euler (ROS)/3(yaw_rad) -> Gain2/1, Mux2/3
  Mux2/1 -> Attitude Controller/7(Orientation roll-pitch-yaw in rad)
  connections:
  plant/RConn1 -- base/RConn1
  collision/RConn1 -- plant/RConn2

== system uas_main_latest/receive position ==
  Bus Selector : BusSelector  OutputSignals=Pose.Position.X,Pose.Position.Y,Pose.Position.Z
  Mux : Mux  Inputs=3
  Subscribe1 : ros2lib/Subscribe  topicSource=Select from ROS network  topic=/cf231/pose  messageType=geometry_msgs/PoseStamped  sampleTime=-1  QOSHistory=Keep last  QOSDepth=1  QOSReliability=Reliable  QOSDurability=Volatile  QOSDeadline=Inf  QOSLifespan=Inf  QOSLiveliness=Automatic  QOSLeaseDuration=Inf  QOSAvoidROSNamespaceConventions=off
  Terminator5 : Terminator
  position : Outport
  wires:
  Subscribe1/2 -> Bus Selector/1
  Mux/1 -> position/1
  Bus Selector/3 -> Mux/3  "<Z>"
  Bus Selector/1 -> Mux/1  "<X>"
  Bus Selector/2 -> Mux/2  "<Y>"
  Subscribe1/1 -> Terminator5/1

== system uas_main_latest/receive setpoint position ==
  Bus Selector : BusSelector  OutputSignals=Position.X,Position.Y,Position.Z
  Mux : Mux  Inputs=3
  Subscribe : ros2lib/Subscribe  topicSource=Specify your own  topic=/cf231/cmd_position  messageType=crazyflie_interfaces/Position  sampleTime=-1  QOSHistory=Keep last  QOSDepth=1  QOSReliability=Reliable  QOSDurability=Volatile  QOSDeadline=Inf  QOSLifespan=Inf  QOSLiveliness=Automatic  QOSLeaseDuration=Inf  QOSAvoidROSNamespaceConventions=off
  Terminator5 : Terminator
  setpoint_position : Outport
  wires:
  Subscribe/2 -> Bus Selector/1
  Mux/1 -> setpoint_position/1
  Bus Selector/3 -> Mux/3  "<Z>"
  Bus Selector/1 -> Mux/1  "<X>"
  Bus Selector/2 -> Mux/2  "<Y>"
  Subscribe/1 -> Terminator5/1

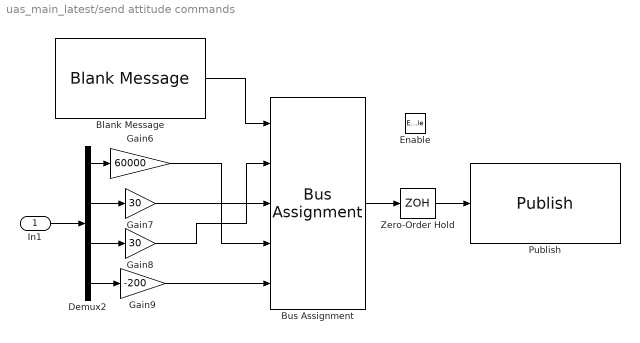
== system uas_main_latest/send attitude commands ==
  In1 : Inport
  Enable : EnablePort
  Blank Message : ros2lib/Blank Message  messageClass=Message  entityType=geometry_msgs/Twist  messageType=geometry_msgs/Twist  SampleTime=inf
  Bus Assignment : BusAssignment  AssignedSignals=Linear.X,Linear.Y,Linear.Z,Angular.Z
  Demux2 : Demux
  Gain6 : Gain  Gain=60000
  Gain7 : Gain  Gain=30
  Gain8 : Gain  Gain=30
  Gain9 : Gain  Gain=-200
  Publish : ros2lib/Publish  topicSource=Specify your own  topic=/cf5/cmd_vel_legacy  messageType=geometry_msgs/Twist  QOSHistory=Keep last  QOSDepth=1  QOSReliability=Reliable  QOSDurability=Volatile  QOSDeadline=Inf  QOSLifespan=Inf  QOSLiveliness=Automatic  QOSLeaseDuration=Inf  QOSAvoidROSNamespaceConventions=off
  Zero-Order Hold : ZeroOrderHold  SampleTime=1/25
  wires:
  Zero-Order Hold/1 -> Publish/1
  Blank Message/1 -> Bus Assignment/1
  Bus Assignment/1 -> Zero-Order Hold/1
  In1/1 -> Demux2/1
  Demux2/1 -> Gain6/1
  Demux2/2 -> Gain7/1
  Demux2/3 -> Gain8/1
  Demux2/4 -> Gain9/1
  Gain6/1 -> Bus Assignment/4
  Gain7/1 -> Bus Assignment/3
  Gain8/1 -> Bus Assignment/2
  Gain9/1 -> Bus Assignment/5

== system uas_main_latest/send setpoint position ==
  p : Inport
  Enable : EnablePort
  send setpoint position : Subsystem
  wires:
  p/1 -> send setpoint position/1(p)

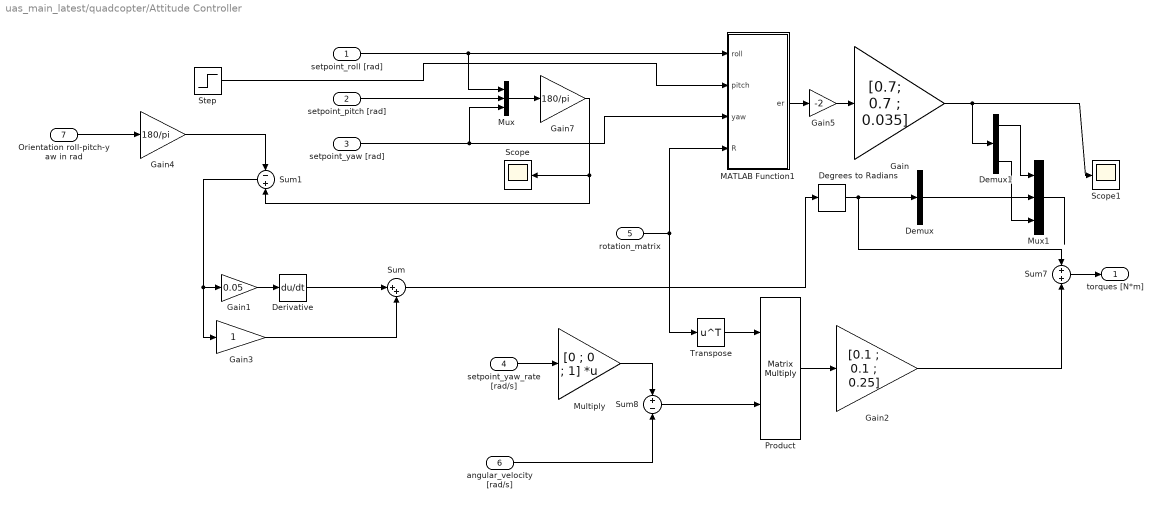
== system uas_main_latest/quadcopter/Attitude Controller ==
  setpoint_roll [rad] : Inport
  setpoint_pitch [rad] : Inport  Port=2
  setpoint_yaw [rad] : Inport  Port=3
  setpoint_yaw_rate [rad/s] : Inport  Port=4
  rotation_matrix : Inport  Port=5
  angular_velocity [rad/s] : Inport  Port=6
  Orientation roll-pitch-yaw in rad : Inport  Port=7
  Degrees to Radians : simulink_extras/Transformations/Degrees to Radians
  Demux : Demux  Outputs=3
  Demux1 : Demux  Outputs=3
  Derivative : Derivative
  Gain : Gain  Gain=[0.7; 0.7 ; 0.035]
  Gain1 : Gain  Gain=0.05
  Gain2 : Gain  Gain=[0.1 ; 0.1 ; 0.25]
  Gain3 : Gain
  Gain4 : Gain  Gain=180/pi
  Gain5 : Gain  Gain=-2
  Gain7 : Gain  Gain=180/pi
  MATLAB Function1 : MATLAB Function  TreatAsAtomicUnit=on
  Multiply : Gain  Gain=[0 ; 0 ; 1]  Multiplication=Matrix(K*u)
  Mux : Mux  Inputs=3
  Mux1 : Mux  Inputs=3
  Product : Product  Multiplication=Matrix(*)
  Scope : Scope
      settings: ActiveDisplayYMinimum=-1  ActiveDisplayYMaximum=1  DataLoggingVariableName=ScopeData5
  Scope1 : Scope
      settings: ActiveDisplayYMinimum=-1  ActiveDisplayYMaximum=1  DataLoggingVariableName=ScopeData7
  Step : Step  Time=0  After=30/180*pi  SampleTime=0
  Sum : Sum  Inputs=|++
  Sum1 : Sum  Inputs=-|+
  Sum7 : Sum
  Sum8 : Sum  Inputs=+|-
  Transpose : Math  Operator=transpose
  torques [N*m] : Outport
  wires:
  setpoint_roll [rad]/1 -> MATLAB Function1/1(roll), Mux/1
  Multiply/1 -> Sum8/1
  Sum8/1 -> Product/2
  Gain2/1 -> Sum7/2
  Gain5/1 -> Gain/1
  setpoint_pitch [rad]/1 -> Mux/2
  angular_velocity [rad/s]/1 -> Sum8/2
  rotation_matrix/1 -> MATLAB Function1/4(R), Transpose/1
  Product/1 -> Gain2/1
  setpoint_yaw_rate [rad/s]/1 -> Multiply/1
  Transpose/1 -> Product/1
  Gain/1 -> Scope1/1, Demux1/1
  MATLAB Function1/1(er) -> Gain5/1
  setpoint_yaw [rad]/1 -> MATLAB Function1/3(yaw), Mux/3
  Sum7/1 -> torques [N*m]/1
  Gain1/1 -> Derivative/1
  Derivative/1 -> Sum/1
  Gain3/1 -> Sum/2
  Sum/1 -> Degrees to Radians/1
  Mux/1 -> Gain7/1
  Orientation roll-pitch-yaw in rad/1 -> Gain4/1
  Gain7/1 -> Sum1/2, Scope/1
  Gain4/1 -> Sum1/1
  Sum1/1 -> Gain3/1, Gain1/1
  Step/1 -> MATLAB Function1/2(pitch)
  Demux1/1 -> Mux1/1
  Demux1/3 -> Mux1/3
  Mux1/1 -> ?
  Demux/2 -> Mux1/2
  Degrees to Radians/1 -> Demux/1, Sum7/1

== system uas_main_latest/quadcopter/mixer ==
  In1 : Inport
  Gain5 : Gain  Gain=mix_matrix  Multiplication=Matrix(K*u)
  Saturation : Saturate  UpperLimit=max_rot_velocity^2  LowerLimit=0
  Sqrt : Sqrt
  Out1 : Outport
  wires:
  Saturation/1 -> Sqrt/1
  In1/1 -> Gain5/1
  Sqrt/1 -> Out1/1
  Gain5/1 -> Saturation/1
